simulink model "mass_spring_damper_PD_controller"  (R2015a)
settings: Solver=ode45  StartTime=0.0  StopTime=60  RelTol=1e-3
undefined symbols (not defined in the file or in its folder): AP, drawMassSpringDamper
settings Model: Creator=ecestudent  LastModifiedBy=wynn4

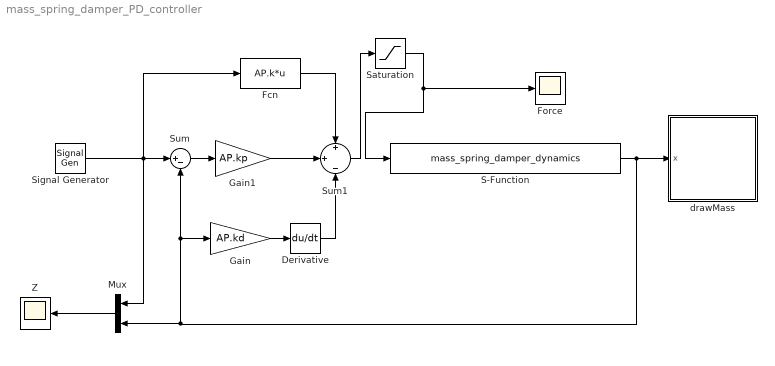
== system mass_spring_damper_PD_controller ==
  Derivative : Derivative
  Fcn : Fcn  Expr=AP.k*u
  Force : Scope
  Gain : Gain  Gain=AP.kd
  Gain1 : Gain  Gain=AP.kp
  Mux : Mux  Inputs=2
  S-Function : S-Function  FunctionName=mass_spring_damper_dynamics  Parameters=AP
  Saturation : Saturate  UpperLimit=2  LowerLimit=-2
  Signal Generator : SignalGenerator  WaveForm=square  Amplitude=.5  Frequency=.02
  Sum : Sum  Inputs=|+-
  Sum1 : Sum  Inputs=+|+|-
  Z : Scope
  drawMass : Subsystem
      mask Display: image(imread('tv.jpg'))
  wires:
  S-Function/1 -> Mux/2, Sum/2, Gain/1, drawMass/1(x)
  Sum/1 -> Gain1/1
  Gain/1 -> Derivative/1
  Signal Generator/1 -> Fcn/1, Mux/1, Sum/1
  Derivative/1 -> Sum1/3
  Gain1/1 -> Sum1/2
  Mux/1 -> Z/1
  Fcn/1 -> Sum1/1
  Sum1/1 -> Saturation/1
  Saturation/1 -> Force/1, S-Function/1

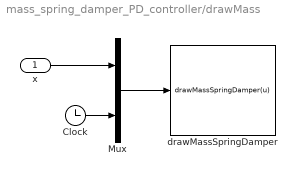
== system mass_spring_damper_PD_controller/drawMass ==
  x : Inport
  Clock : Clock
  Mux : Mux  Inputs=2
  drawMassSpringDamper : MATLABFcn  MATLABFcn=drawMassSpringDamper(u)  OutputDimensions=0
      mask Display: image(imread('tv.jpg'))
  wires:
  x/1 -> Mux/1
  Clock/1 -> Mux/2
  Mux/1 -> drawMassSpringDamper/1
